simulink model "FM_Bistatic_Radar_V2"  (R2025a)
settings: Solver=VariableStepAuto  StartTime=0.0  StopTime=10.0  RelTol=1e-3
undefined symbols (not defined in the file): physconst
libraries: commchan3 x2, phaseddetectlib x2, dspadpt3 x1, phasedenvlib x1, dspmlti4 x1, dspxfrm3 x1
settings Model: Creator=leifefrancisco  LastModifiedBy=leifefrancisco

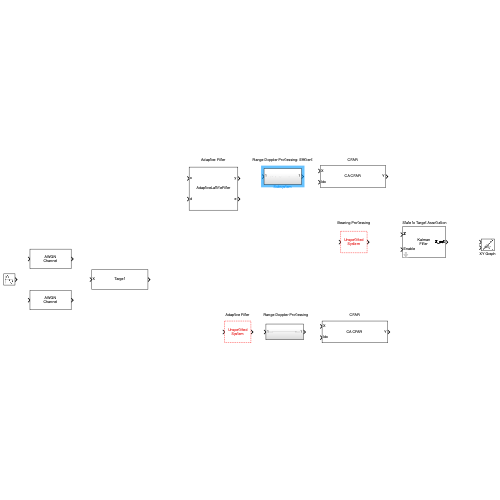
[thumbnail: Simulink's stored preview of the top-level diagram]
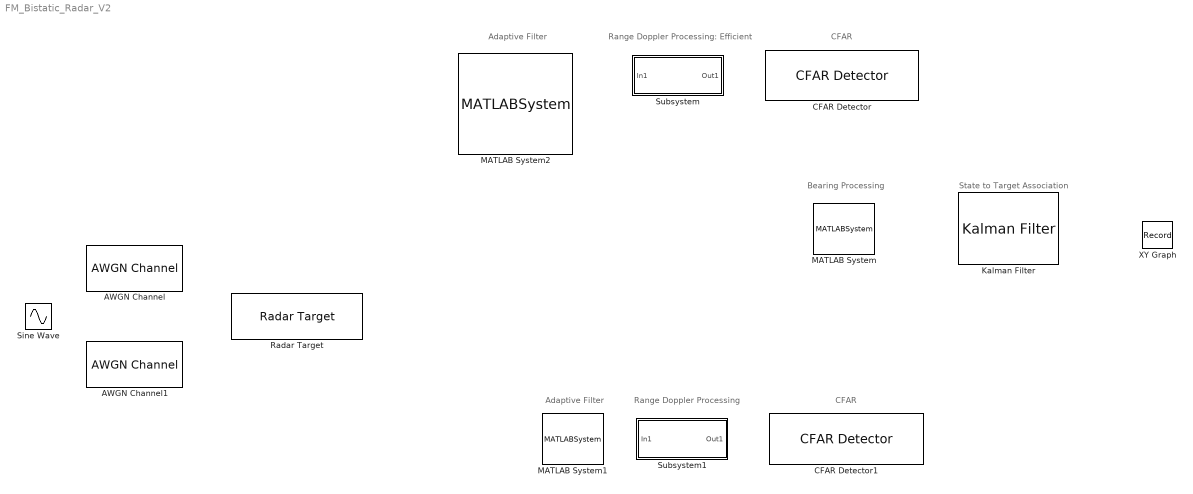
== system FM_Bistatic_Radar_V2 ==
  note: State to Target Association
  note: Bearing Processing
  note: CFAR
  note: Range Doppler Processing: Efficient
  note: Adaptive Filter
  note: Range Doppler Processing
  note: CFAR
  note: Adaptive Filter
  AWGN Channel : commchan3/AWGN Channel  LegacyMode=off  NoiseMethod="Signal to noise ratio  (SNR)"  noiseMode="Signal to noise ratio  (SNR)"  EbNo=10  EsNo=10  SNR=10  BitsPerSymbol=1  SignalPower=1  SpecifySymbolPeriod=off  SamplesPerSymbol=1  SymbolPeriod=1  VarianceSource=Parameter  Variance=1  RandomStream=Global stream  Seed=67  SimulateUsing=Code generation
  AWGN Channel1 : commchan3/AWGN Channel  LegacyMode=off  NoiseMethod="Signal to noise ratio  (SNR)"  noiseMode="Signal to noise ratio  (SNR)"  EbNo=10  EsNo=10  SNR=10  BitsPerSymbol=1  SignalPower=1  SpecifySymbolPeriod=off  SamplesPerSymbol=1  SymbolPeriod=1  VarianceSource=Parameter  Variance=1  RandomStream=Global stream  Seed=67  SimulateUsing=Code generation
  CFAR Detector : phaseddetectlib/CFAR Detector  Method=CA  Rank=1  NumGuardCells=2  NumTrainingCells=2  ThresholdFactor=Auto  ProbabilityFalseAlarm=0.1  CustomThresholdFactor=1  OutputFormat=CUT result  ThresholdOutputPort=off  NoisePowerOutputPort=off  NumDetectionsSource=Auto  NumDetections=1  SimulateUsing=Interpreted execution
  CFAR Detector1 : phaseddetectlib/CFAR Detector  Method=CA  Rank=1  NumGuardCells=2  NumTrainingCells=2  ThresholdFactor=Auto  ProbabilityFalseAlarm=0.1  CustomThresholdFactor=1  OutputFormat=CUT result  ThresholdOutputPort=off  NoisePowerOutputPort=off  NumDetectionsSource=Auto  NumDetections=1  SimulateUsing=Interpreted execution
  Kalman Filter : dspadpt3/Kalman Filter  num_targets=10  sourceEnable=Specify via input port <Enable>  isReset=on  X=zeros([6, 1])  P=10*eye(6)  A=[1 0 1 0 0 0;0 1 0 1 0 0; 0 0 1 0 0 0; 0 0 0 1 0 0; 0 0 0 0 1 0; 0 0 0 0 0 1]  sourceMeasure=Specify via dialog  H=[1 0 0 0 0 0; 0 1 0 0 0 0; 0 0 0 0 1 0; 0 0 0 0 0 1]  Q=0.05*eye(6)  R=eye(4)  isOutputEstMeasure=on  isOutputEstState=off  isOutputEstError=off  isOutputPrdMeasure=off  isOutputPrdState=off  isOutputPrdError=off
  MATLAB System : MATLABSystem
  MATLAB System1 : MATLABSystem
  MATLAB System2 : MATLABSystem  System=dsp.AdaptiveLatticeFilter  Method=Least-squares Lattice  Length=32  ForgettingFactor=1  StepSize=0.1  ReflectionStepSize=0.1  AveragingFactor=0.9  InitialPredictionErrorPower=1  InitialCoefficients=0  LockCoefficients=off  SimulateUsing=Code generation  Offset=1
      mask Type: dsp.AdaptiveLatticeFilter
  Radar Target : phasedenvlib/Radar Target  EnablePolarization=off  Mode=Monostatic  MeanRCSSource=Property  ScatteringMatrixSource=Property  MeanRCS=1  ScatteringMatrix=eye( 2 )  Model=Nonfluctuating  PropagationSpeed=physconst( 'LightSpeed' )  OperatingFrequency=3e8  SeedSource=Auto  Seed=0  SimulateUsing=Interpreted execution
  Sine Wave : Sin  SampleTime=0
  Subsystem : Subsystem
  Subsystem1 : Subsystem
  XY Graph : Record  NumPorts=2.0  FileSettingsInternal="{\"entries\":[{\"content\":{\"excelSettings\":{\"content\":{},\"type\":\"Streamout.ExcelSettings\"},\"parquetSettings\":{\"content\":{},\"type\":\"Streamout.ParquetSettings\"}},\"type\":\"Streamout.FileSettingStorage\",\"uuid\":\"\"}],\"packageUris\":[\"http:\\/\\/schema.mathworks.com\\/mf0\\/streamout_blocks\\/R2020a\"],\"version\":\"1.0\"}"  FrameSettings=[0, 0]  Layout=[1 1]  SignalsInternal="{\"entries\":[{\"content\":{\"signals\":[{\"content\":{\"blockPath\":[],\"dimensions\":[1],\"domain\":\"\",\"lineColor\":\"#a2142f\",\"plots\":[ 1 ],\"port\":1,\"signalID\":1,\"signalName\":\"XY Graph:1\"},\"type\":\"RecordBlkView.Signal\",\"uuid\":\"\"},{\"content\":{\"blockPath\":[],\"dimensions\":[1],\"domain\":\"\",\"lineColor\":\"#139fff\",\"plots\":[ 1 ],\"port\":2,\"signalID\":2,\"signalName\":\"XY Graph:2\"},\"type\":\"RecordBlkView.Signal\",\"uuid\":\"\"}]},\"type\":\"RecordBlkView.InputSignals\",\"uuid\":\"\"}],\"packageUris\":[\"http:\\/\\/schema.mathworks.com\\/mf0\\/streamout_blocks\\/R2020a\"],\"version\":\"1.0\"}"  VisualizationBindings="{\"xyplotplugin\":{\"info\":[{\"series\":[{\"bindingParametersList\":[{\"parameter\":\"X-Axis\",\"signalID\":1,\"signalName\":\"XY Graph:1\"},{\"parameter\":\"Y-Axis\",\"signalID\":2,\"signalName\":\"XY Graph:2\"}],\"seriesID\":0}],\"subplotID\":1}]}}"  CompatibilityTag=XY

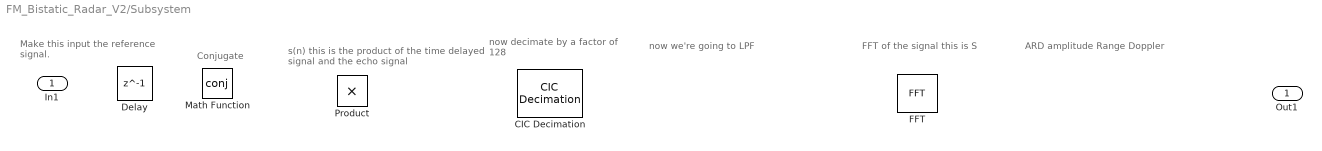
== system FM_Bistatic_Radar_V2/Subsystem ==
  note: Make this input the reference
      | signal.
  note: ARD amplitude Range Doppler
  note: FFT of the signal this is S
  note: now we're going to LPF
  note: now decimate by a factor
      | of 128
  note: s(n) this is the product of the
      | time delayed signal and the echo signal
  note: Conjugate
  In1 : Inport
  CIC Decimation : dspmlti4/CIC Decimation  filtFrom=Dialog parameters  filtobj=CICDECIM  ftype=Decimator  R=2  M=1  N=2  filterInternals=Full precision  BPS=[16 16 16 16]  FLPS=0  outputWordLength=32  outputFracLength=0  launchFVT=off  framing=Maintain input frame rate  RateOptions=Enforce single-rate processing
  Delay : Delay  DelayLength=1  InitialCondition=0
  FFT : dspxfrm3/FFT  FFTImplementation=Auto  CompMethod=Table lookup  TableOpt=NEW  TableOptActive=Speed  BitRevOrder=off  Normalize=off  InheritFFTLength=on  FFTLength=64  WrapInput=on  roundingMode=Ceiling  overflowMode=off  firstCoeffDataTypeStr=Inherit: Same word length as input  firstCoeffLastDataTypeStr=Inherit: Same word length as input  outputMin=[]  outputMax=[]
  Math Function : Math  Operator=conj
  Product : Product
  Out1 : Outport

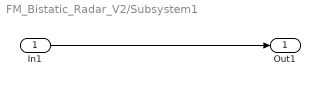
== system FM_Bistatic_Radar_V2/Subsystem1 ==
  In1 : Inport
  Out1 : Outport
  wires:
  In1/1 -> Out1/1
